simulink model "Lecture28sim"  (R2018a)
settings: Solver=VariableStepAuto  StartTime=0.0  StopTime=2  RelTol=1e-3
values from neighbouring files (symbols this model uses):
  A = [0,1;16,0]    [Lecture24.m]    (also in Lecture27.m; Lecture28.m = [ 0   1   0; Lecture28simulink.m = [ 0   1   0; solveACmx.m = input('Enter A matrix now (must be n x n): '))
  B = [0;1]    [Lecture24.m]    (also in Lecture27.m; Lecture28.m = [ 0; Lecture28simulink.m = [ 0; solveACmx.m = input('Enter B matrix now (must be n x 1): '))
  C = [1,0]    [Lecture24.m]    (also in Lecture27.m; Lecture28.m = [ 1 0 0 ]; Lecture28simulink.m = [ 1 0 0 ])
  K1 = K(1)    [Lecture28simulink.m]
  K2 = K(2)    [Lecture28simulink.m]
  K3 = K(3)    [Lecture28simulink.m]
  Nbar = rscale(sys,K)    [Lecture28.m]    (also in Lecture28simulink.m)
libraries: cstblocks x1
settings Model: Creator=b.mcpheron  LastModifiedBy=b.mcpheron

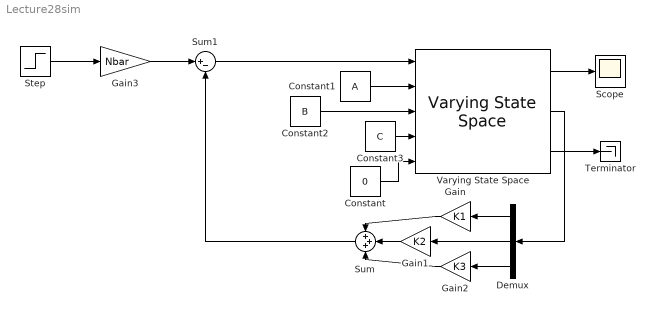
== system Lecture28sim ==
  Constant : Constant  Value=0
  Constant1 : Constant  Value=A  VectorParams1D=off
  Constant2 : Constant  Value=B  VectorParams1D=off
  Constant3 : Constant  Value=C  VectorParams1D=off
  Demux : Demux  Outputs=3
  Gain : Gain  Gain=K1
  Gain1 : Gain  Gain=K2
  Gain2 : Gain  Gain=K3
  Gain3 : Gain  Gain=Nbar
  Scope : Scope
  Step : Step  Time=0  SampleTime=0
  Sum : Sum  Inputs=+++
  Sum1 : Sum  Inputs=|+-
  Terminator : Terminator
  Varying State Space : cstblocks/Linear Parameter Varying/Varying State Space  x0=0  xNames=''  OutputX=on  OutputDX=on
      settings: SourceProductName=Control System Toolbox
  wires:
  Constant1/1 -> Varying State Space/2
  Constant2/1 -> Varying State Space/3
  Constant3/1 -> Varying State Space/4
  Constant/1 -> Varying State Space/5
  Demux/1 -> Gain/1
  Demux/2 -> Gain1/1
  Demux/3 -> Gain2/1
  Varying State Space/2 -> Demux/1
  Gain1/1 -> Sum/2
  Gain/1 -> Sum/1
  Gain2/1 -> Sum/3
  Sum1/1 -> Varying State Space/1
  Sum/1 -> Sum1/2
  Varying State Space/1 -> Scope/1
  Step/1 -> Gain3/1
  Gain3/1 -> Sum1/1
  Varying State Space/3 -> Terminator/1
